simulink model "SC_RL_eval"  (R2021a)
settings: Solver=FixedStepAuto  StartTime=0.0  StopTime=T  FixedStep=Ts  MaxStep=0.1  RelTol=1e-3  EnableMultiTasking=on
PreLoadFcn:
  | K=10.8;
  | TI=2.56;
  | TD=0;
  | u=0;
InitFcn:
  | seed = randi(10000);
StartFcn:
  | seed = randi(10000);
undefined symbols (not defined in the file): isTerminate, P_final, P_init, P_step, P_terminate
libraries: simulink x3, simulink_extras x2, rllib x1
settings Model: Creator=jiaya  LastModifiedBy=jiaya
settings SolverCC: AlgebraicLoopSolver=TrustRegion
settings DataIOCC: LimitDataPoints=on  SaveFormat=Array  SignalLoggingSaveFormat=ModelDataLogs  ReturnWorkspaceOutputs=off
settings OptimizationCC: InitFltsAndDblsToZero=on  LifeSpan=inf
settings DebuggingCC: SaveWithParameterizedLinksMsg=none  UnderspecifiedInitializationDetection=Classic  MergeDetectMultiDrivingBlocksExec=none  SignalResolutionControl=TryResolveAllWithWarning  MultiTaskDSMMsg=warning  MultiTaskCondExecSysMsg=none  FcnCallInpInsideContextMsg=warning  SFUnexpectedBacktrackingDiag=warning  SFNoUnconditionalDefaultTransitionDiag=warning  SFExecutionAtInitializationDiag=none  SFMachineParentedDataDiag=warning  ArithmeticOperatorsInVariantConditions=warning
settings HardwareCC: ProdBitPerPointer=32  ProdBitPerSizeT=32  ProdBitPerPtrDiffT=32  ProdLargestAtomicFloat=None  ProdIntDivRoundTo=Undefined  ProdEndianess=Unspecified  ProdWordSize=32  ProdHWDeviceType=32-bit Generic  TargetUnknown=on
settings ModelReferenceCC: PropagateSignalLabelsOutOfModel=off
settings CodeAppCC: StateflowObjectComments=on
settings GRTTargetCC: TargetFcnLib=ansi_tfl_tmw.mat  TargetLangStandard=C89/C90 (ANSI)  CombineOutputUpdateFcns=off  GRTInterface=on
settings ConfigComp: CovMetricSettings=dw  CovSaveCumulativeToWorkspaceVar=on  CovSaveSingleToWorkspaceVar=on

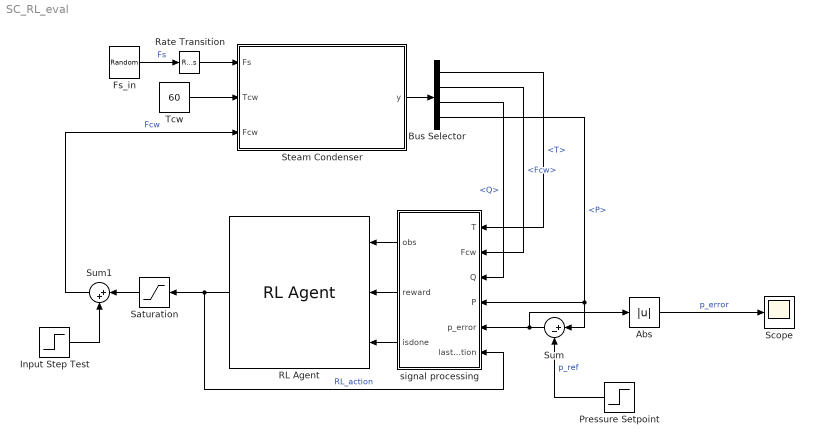
== system SC_RL_eval ==
  Abs : Abs
  Bus Selector : BusSelector  OutputSignals=T,Fcw,Q,P
  Fs_in : UniformRandomNumber  Minimum=3.99  Maximum=4.01  Seed=seed  SampleTime=5  VectorParams1D=off
  Input Step Test : Step  Time=10  After=0  SampleTime=0
  Pressure Setpoint : Step  Time=P_step  Before=P_init  After=P_final  SampleTime=0
  RL Agent : rllib/RL Agent  Agent=agent  ExternalActionAsInput=off  ProvideCumRwd=off  TreatAsDirectFeedthrough=on
  Rate Transition : RateTransition  OutPortSampleTime=Ts
  Saturation : Saturate  UpperLimit=500  LowerLimit=-1200
  Scope : Scope
  Steam Condenser : Subsystem  mask{V=3, Mcw=500, UA=356.972413581334, tau=1, Fcw=107.8880952381, P=90, T=80}
      mask prompts: V "Volume [m3]"; Mcw "CW Holdup [kg]"; UA "UA [kW/K]"; tau "Actuator time constant [s]"; Fcw "Fcw [kg/s]"; P "P [kPa]"; T "T [degC]"
      mask init:
      | y1=[.3 .3 .7 .7 .3 NaN .4 .4 NaN .5 .5 NaN .6 .6 NaN 0.2 0.3 NaN 0.7 0.8 NaN 0.7 0.8 NaN 0.82 NaN 0.18];
      | x1=[.8 .2 .2 .8 .8 NaN .8 .2 NaN .8 .2 NaN .8 .2 NaN 0.5 0.5 NaN 0.3 0.3 NaN 0.7 0.7 NaN -0.05 NaN 1.05];
      | y2=0.3:0.05:0.7;
      | x2=sqrt(0.0625-(y2-0.5).^2);
      | y3=[.5 .5 .8 NaN 0.2 0.4 0.4];
      | x3=[x2(5)+0.65 0.95 0.95 NaN .1 .1 0.35-x2(3)];
      mask Display:
      | plot([x1 NaN 0.65+x2 NaN 0.35-x2 NaN x3],[y1 NaN y2 NaN y2 NaN y3])
      | port_label('input',1,'Fs')
      | port_label('input',2,'Tcw')
      | port_label('input',3,'Fcw')
      | port_label('output',1,'y')
  Sum : Sum  Inputs=|+-  InputSameDT=on  OutDataTypeStr=Inherit: Same as first input
  Sum1 : Sum  Inputs=|++  InputSameDT=on  OutDataTypeStr=Inherit: Same as first input
  Tcw : Constant  Value=60  VectorParams1D=off
  signal processing : Subsystem
  wires:
  Steam Condenser/1(y) -> Bus Selector/1
  Tcw/1 -> Steam Condenser/2(Tcw)
  Pressure Setpoint/1 -> Sum/2  "p_ref"
  Bus Selector/1 -> signal processing/1(T)  "<T>"
  Bus Selector/2 -> signal processing/2(Fcw)  "<Fcw>"
  Bus Selector/3 -> signal processing/3(Q)  "<Q>"
  Bus Selector/4 -> Sum/1, signal processing/4(P)  "<P>"
  Sum1/1 -> Steam Condenser/3(Fcw)  "Fcw"
  Input Step Test/1 -> Sum1/2
  Fs_in/1 -> Rate Transition/1  "Fs"
  signal processing/1(obs) -> RL Agent/1
  signal processing/2(reward) -> RL Agent/2
  signal processing/3(isdone) -> RL Agent/3
  Sum/1 -> Abs/1, signal processing/5(p_error)
  RL Agent/1 -> signal processing/6(last_action), Saturation/1  "RL_action"
  Rate Transition/1 -> Steam Condenser/1(Fs)
  Saturation/1 -> Sum1/1
  Abs/1 -> Scope/1  "p_error"

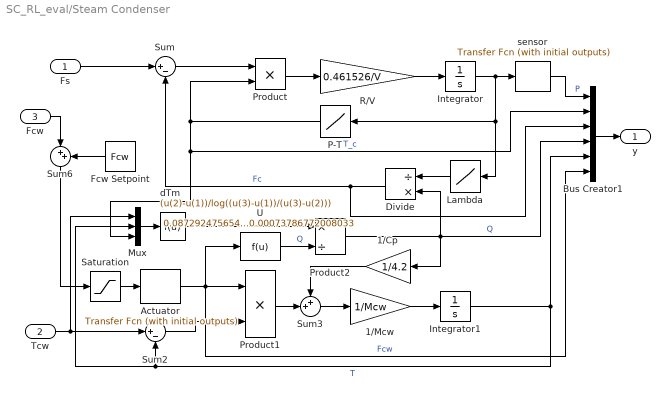
== system SC_RL_eval/Steam Condenser ==
  Fs : Inport
  Tcw : Inport  Port=2
  Fcw : Inport  Port=3
  1/Cp : Gain  Gain=1/4.2  OutDataTypeStr=Inherit: Same as input  ParamDataTypeStr=Inherit: Same as input
  1/Mcw : Gain  Gain=1/Mcw  OutDataTypeStr=Inherit: Same as input  ParamDataTypeStr=Inherit: Same as input
  Actuator : simulink_extras/Additional Linear/Transfer Fcn (with initial outputs)  N=[1]  D=[tau 1]  Y0=Fcw  U0=Fcw
  Bus Creator1 : BusCreator  Inputs=6
  Divide : Product  Inputs=/*  InputSameDT=on  RndMeth=Zero  OutDataTypeStr=Inherit: Same as first input
  Fcw Setpoint : Constant  Value=Fcw
  Integrator : Integrator  InitialCondition=P
  Integrator1 : Integrator  InitialCondition=T
  Lambda : Lookup  InputValues=[50 60 70 80 90 100 110]  Table=[2305.42 2293.64 2283.30 2274.05 2265.65 2257.92 2250.76]  SaturateOnIntegerOverflow=on
  Mux : Mux  Inputs=3
  P-T : Lookup  InputValues=[50 60 70 80 90 100 110]  Table=[81.3167 85.9258 89.9315 93.4854 96.6870 99.6059 102.2923]  SaturateOnIntegerOverflow=on
  Product : Product  InputSameDT=on  RndMeth=Zero  OutDataTypeStr=Inherit: Same as first input
  Product1 : Product  InputSameDT=on  RndMeth=Zero  OutDataTypeStr=Inherit: Same as first input
  Product2 : Product  Inputs=*/  InputSameDT=on  RndMeth=Zero  OutDataTypeStr=Inherit: Same as first input
  R/V : Gain  Gain=0.461526/V  OutDataTypeStr=Inherit: Same as input  ParamDataTypeStr=Inherit: Same as input
  Saturation : Saturate  UpperLimit=200  LowerLimit=0
  Sum : Sum  Inputs=|+-  InputSameDT=on  OutDataTypeStr=Inherit: Same as first input
  Sum2 : Sum  Inputs=|+-  InputSameDT=on  OutDataTypeStr=Inherit: Same as first input
  Sum3 : Sum  Inputs=++|  InputSameDT=on  OutDataTypeStr=Inherit: Same as first input
  Sum6 : Sum  Inputs=|++  InputSameDT=on  OutDataTypeStr=Inherit: Same as first input
  U : Fcn  Expr=0.0872924756541668/u^0.8+0.00073786772008033
  dTm : Fcn  Expr=(u(2)-u(1))/log((u(3)-u(1))/(u(3)-u(2)))
  sensor : simulink_extras/Additional Linear/Transfer Fcn (with initial outputs)  N=[1]  D=[tau/2 1]  Y0=P  U0=P
  y : Outport
  wires:
  R/V/1 -> Integrator/1
  Product/1 -> R/V/1
  Sum/1 -> Product/1
  Fs/1 -> Sum/1
  Integrator/1 -> sensor/1, Lambda/1, P-T/1
  1/Mcw/1 -> Integrator1/1
  Integrator1/1 -> Sum2/2, Mux/2, Bus Creator1/5  "T"
  Tcw/1 -> Sum2/1, Mux/1
  Sum2/1 -> Product1/2
  Product1/1 -> Sum3/2
  Sum3/1 -> 1/Mcw/1
  1/Cp/1 -> Sum3/1
  dTm/1 -> Product2/1
  Bus Creator1/1 -> y/1
  Actuator/1 -> Product1/1, U/1, Bus Creator1/6  "Fcw"
  sensor/1 -> Bus Creator1/1  "P"
  Saturation/1 -> Actuator/1
  Sum6/1 -> Saturation/1
  Fcw/1 -> Sum6/1
  Fcw Setpoint/1 -> Sum6/2
  Lambda/1 -> Divide/1
  Divide/1 -> Sum/2, Bus Creator1/3  "Fc"
  P-T/1 -> Product/2, Mux/3, Bus Creator1/2  "T_c"
  Mux/1 -> dTm/1
  Product2/1 -> 1/Cp/1, Divide/2, Bus Creator1/4  "Q"
  U/1 -> Product2/2  "Q"

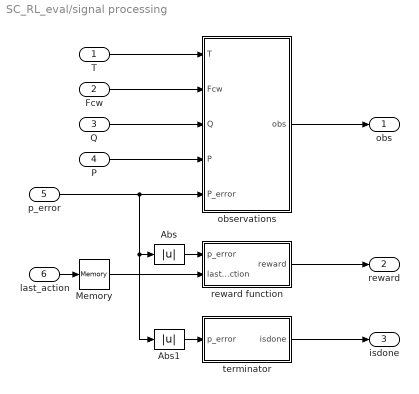
== system SC_RL_eval/signal processing ==
  T : Inport
  Fcw : Inport  Port=2
  Q : Inport  Port=3
  P : Inport  Port=4
  p_error : Inport  Port=5
  last_action : Inport  Port=6
  Abs : Abs
  Abs1 : Abs
  Memory : Memory
  observations : Subsystem
  reward function : Subsystem
  "terminator " : Subsystem
  obs : Outport
  reward : Outport  Port=2
  isdone : Outport  Port=3
  wires:
  T/1 -> observations/1(T)
  Fcw/1 -> observations/2(Fcw)
  Q/1 -> observations/3(Q)
  P/1 -> observations/4(P)
  observations/1(obs) -> obs/1
  reward function/1(reward) -> reward/1
  "terminator "/1(isdone) -> isdone/1
  p_error/1 -> observations/5(P_error), Abs/1, Abs1/1
  last_action/1 -> Memory/1
  Memory/1 -> reward function/2(last_action)
  Abs/1 -> reward function/1(p_error)
  Abs1/1 -> "terminator "/1(p_error)

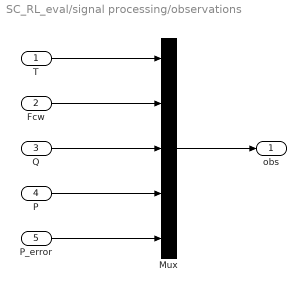
== system SC_RL_eval/signal processing/observations ==
  T : Inport
  Fcw : Inport  Port=2
  Q : Inport  Port=3
  P : Inport  Port=4
  P_error : Inport  Port=5
  Mux : Mux  Inputs=5
  obs : Outport
  wires:
  Mux/1 -> obs/1
  T/1 -> Mux/1
  Fcw/1 -> Mux/2
  Q/1 -> Mux/3
  P/1 -> Mux/4
  P_error/1 -> Mux/5

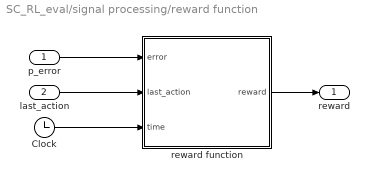
== system SC_RL_eval/signal processing/reward function ==
  p_error : Inport
  last_action : Inport  Port=2
  Clock : Clock
  reward function : MATLAB Function  TreatAsAtomicUnit=on
  reward : Outport
  wires:
  reward function/1(reward) -> reward/1
  p_error/1 -> reward function/1(error)
  last_action/1 -> reward function/2(last_action)
  Clock/1 -> reward function/3(time)

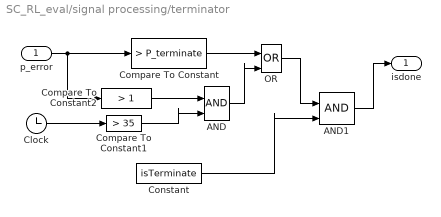
== system SC_RL_eval/signal processing/terminator  ==
  p_error : Inport
  AND : Logic  IconShape=distinctive  AllPortsSameDT=off  OutDataTypeStr=boolean
  AND1 : Logic  IconShape=distinctive  AllPortsSameDT=off  OutDataTypeStr=boolean
  Clock : Clock
  Compare To Constant : simulink/Logic and Bit Operations/Compare To Constant  relop=>  const=P_terminate  OutDataTypeStr=boolean
  Compare To Constant1 : simulink/Logic and Bit Operations/Compare To Constant  relop=>  const=35  OutDataTypeStr=boolean
  Compare To Constant2 : simulink/Logic and Bit Operations/Compare To Constant  relop=>  const=1  OutDataTypeStr=boolean
  Constant : Constant  Value=isTerminate
  OR : Logic  Operator=OR  IconShape=distinctive  AllPortsSameDT=off  OutDataTypeStr=boolean
  isdone : Outport
  wires:
  p_error/1 -> Compare To Constant2/1, Compare To Constant/1
  Compare To Constant/1 -> OR/1
  AND/1 -> OR/2
  Clock/1 -> Compare To Constant1/1
  Compare To Constant2/1 -> AND/1
  Compare To Constant1/1 -> AND/2
  OR/1 -> AND1/1
  AND1/1 -> isdone/1
  Constant/1 -> AND1/2

== matlab function SC_RL_eval/signal processing/reward function/reward function ==
  data: error input; reward output; last_action input; time input
function reward = fcn(error, last_action, time)

% if time < 20
%     reward = -2*tanh(error/15) + 2*exp(-error/10);
% else
%     reward = -5*tanh(error) + 5*exp(-error*1.5);
% end

% if time < 15
%     reward = -0.1*tanh(error/15) + 0.1*exp(-error/10);
% elseif time < 20
%     reward = -1*tanh(error/4) + 1*exp(-error/2);
% else
%         reward = -5*tanh(error) + 5*exp(-error);
% end

reward = -tanh(error);
